simulink model "direction_sim"  (R2023a)
settings: configuration reference "config" (kept outside this file)
model workspace (MATLAB code in the model file + MAT data in the model file):
  cmdLim = Simulink.Parameter
  cmdLim.Value = 15
  cmdLim.Description = 'Limit for controlling the maximum surface command angle.'
  cmdLim.Min = 0
  cmdLim.Max = 90
  cmdLim.DocUnits = 'deg'
  dispGain = Simulink.Parameter
  dispGain.Value = 0.75
  dispGain.Description = 'Gain applied to the displacement error.'
  dispGain.Min = 0
  dispGain.Max = []
  dispGain.DocUnits = 'deg/sec/deg'
  dispLim = Simulink.Parameter
  dispLim.Value = 30
  dispLim.Description = 'Limit for controlling the maximum commanded angle.'
  dispLim.Min = 0
  dispLim.Max = 180
  dispLim.DocUnits = 'deg'
  intGain = Simulink.Parameter
  intGain.Value = 0.5
  intGain.Description = 'Gain applied to the integral error.'
  intGain.Min = 0
  intGain.Max = []
  intGain.DocUnits = 'deg/sec/deg/sec'
  intLim = Simulink.Parameter
  intLim.Value = 5
  intLim.Description = 'Limit for controlling the maximum commanded angle.'
  intLim.Min = 0
  intLim.Max = 90
  intLim.DocUnits = 'deg'
  rateGain = Simulink.Parameter
  rateGain.Value = 2
  rateGain.Description = 'Gain applied to the rate error.'
  rateGain.Min = 0
  rateGain.Max = []
  rateGain.DocUnits = 'deg/deg/sec'
  rateLim = Simulink.Parameter
  rateLim.Value = 6
  rateLim.Description = 'Limit for controlling the maximum commanded angle.'
  rateLim.Min = 0
  rateLim.Max = 180
  rateLim.DocUnits = 'deg/sec'
  hdgGain = Simulink.Parameter
  hdgGain.Value = 0.015
  b = Simulink.Parameter
  b.Value = 0.001
  b.DataType = 'single'
  b.Complexity = 'real'
  b.Dimensions = [1 1]
  enc_line = Simulink.Parameter
  enc_line.Value = 10000
  enc_line.DataType = 'single'
  enc_line.Complexity = 'real'
  enc_line.Dimensions = [1 1]
  fc = Simulink.Parameter
  fc.Value = 0.01
  fc.DataType = 'single'
  fc.Complexity = 'real'
  fc.Dimensions = [1 1]
  flux = Simulink.Parameter
  flux.Value = 0.0125
  flux.DataType = 'single'
  flux.Complexity = 'real'
  flux.Dimensions = [1 1]
  fs = Simulink.Parameter
  fs.Value = 10000
  fs.Description = '位置环 速度环执行频率'
  fs.DataType = 'single'
  fs.Complexity = 'real'
  fs.Dimensions = [1 1]
  j = Simulink.Parameter
  j.Value = 1.9e-05
  j.DataType = 'single'
  j.Complexity = 'real'
  j.Dimensions = [1 1]
  j_inv = Simulink.Parameter
  j_inv.Value = 52631.5789474
  j_inv.DataType = 'single'
  j_inv.Complexity = 'real'
  j_inv.Dimensions = [1 1]
  kt = Simulink.Parameter
  kt.Value = 0.075
  kt.DataType = 'single'
  kt.Complexity = 'real'
  kt.Dimensions = [1 1]
  ld = Simulink.Parameter
  ld.Value = 0.00059
  ld.Description = '定子电感 H'
  ld.DataType = 'single'
  ld.Complexity = 'real'
  ld.Dimensions = [1 1]
  ld_inv = Simulink.Parameter
  ld_inv.Value = 1694.91525424
  ld_inv.Description = '定子电感 H'
  ld_inv.DataType = 'single'
  ld_inv.Complexity = 'real'
  ld_inv.Dimensions = [1 1]
  lq = Simulink.Parameter
  lq.Value = 0.00059
  lq.Description = '定子电感 H'
  lq.DataType = 'single'
  lq.Complexity = 'real'
  lq.Dimensions = [1 1]
  lq_inv = Simulink.Parameter
  lq_inv.Value = 1694.91525424
  lq_inv.Description = '定子电感 H'
  lq_inv.DataType = 'single'
  lq_inv.Complexity = 'real'
  lq_inv.Dimensions = [1 1]
  pn = Simulink.Parameter
  pn.Value = 4
  pn.DataType = 'single'
  pn.Complexity = 'real'
  pn.Dimensions = [1 1]
  r = Simulink.Parameter
  r.Value = 1.02
  r.Description = '定子电阻 ohm'
  r.DataType = 'single'
  r.Complexity = 'real'
  r.Dimensions = [1 1]
  tc = Simulink.Parameter
  tc.Value = 5e-05
  tc.Description = '电流环运行频率用来设定综合仿真的参数'
  tc.DataType = 'double'
  tc.Complexity = 'real'
  tc.Dimensions = [1 1]
  tp = Simulink.Parameter
  tp.Value = 0.0001
  tp.Description = '位置环速度环执行周期'
  tp.DataType = 'double'
  tp.Complexity = 'real'
  tp.Dimensions = [1 1]
  ts = Simulink.Parameter
  ts.Value = 1e-05
  ts.Description = '模型仿真的周期 s'
  ts.DataType = 'double'
  ts.Complexity = 'real'
  ts.Dimensions = [1 1]
libraries: simulink x2
settings Model: RequirementInfo={} %GIDa_fe9045fd_0412_4b6e_8206_617cc20e6fde  DataDictionary=model_config.sldd  ParameterArgumentNames=b,enc_line,fc,flux,fs,j,j_inv,kt,ld,ld_inv,lq,lq_inv,pn,r  Creator=Administrator  LastModifiedBy=Administrator
settings ConfigSetRef: SourceName=config

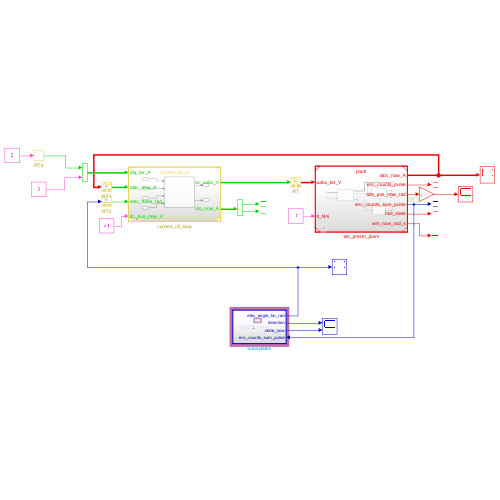
[thumbnail: Simulink's stored preview of the top-level diagram]
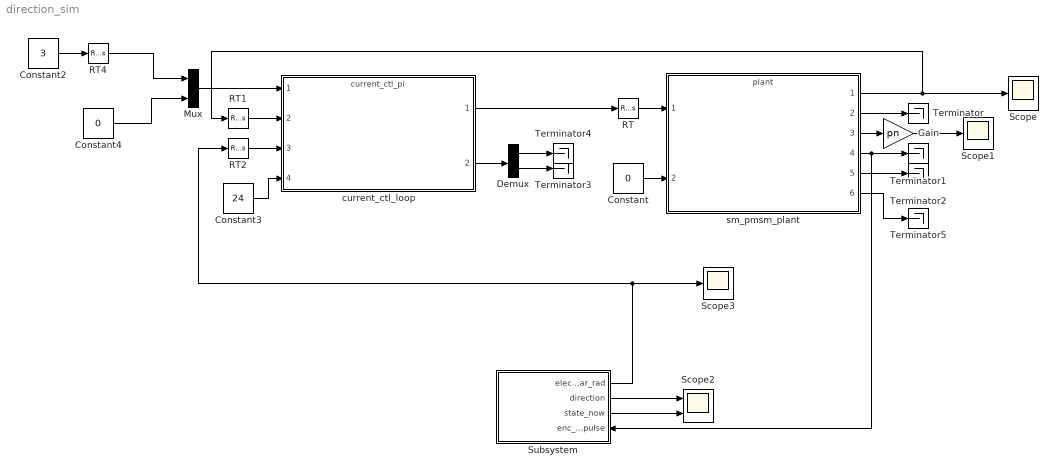
== system direction_sim ==
  Constant : Constant  Value=0  OutDataTypeStr=single
  Constant2 : Constant  Value=3  OutDataTypeStr=single
  Constant3 : Constant  Value=24  OutDataTypeStr=single
  Constant4 : Constant  Value=0  OutDataTypeStr=single
  Demux : Demux  Outputs=2
  Gain : Gain  Gain=pn
  Mux : Mux  Inputs=2
  RT : RateTransition  OutPortSampleTime=ts
  RT1 : RateTransition  OutPortSampleTime=tc
  RT2 : RateTransition  OutPortSampleTime=tc
  RT4 : RateTransition  OutPortSampleTime=tc
  Scope : Scope
  Scope1 : Scope
  Scope2 : Scope  NumInputPorts=2
  Scope3 : Scope
  Subsystem : Subsystem  TreatAsAtomicUnit=on  SystemSampleTime=10e-5
      settings: PortSchema="{\"entries\":[{\"content\":{\"sides\":[{\"content\":{},\"type\":\"ConnectorPlacement.EquallySpacedRectSide\",\"uuid\":\"d07efbd3-f561-406e-a8ff-2cd425a2d2f1\"},{\"content\":{\"connectorIds\":[\"Out1\",\"Out2\",\"Out3\",\"In1\"],\"side\":\"RIGHT\"},\"type\":\"ConnectorPlacement.EquallySpacedRectSide\",\"uuid\":\"8e75d4b6-33a0-42ab-8f9a-b924bdc8bdb3\"},{\"content\":{\"side\":\"TOP\"},\"type\":\"ConnectorPlacement.EquallySpacedRectSide\",\"uuid\":\"05e65f83-a04f-4767-afb8-de784f70a9b2\"}]},\"type\":\"ConnectorPlacement.EquallySpacedConnector\",\"uuid\":\"6847f190-d81b-4cfc-961e-3d73d3d3f65e\"}],\"packageUris\":[\"http://schema.mathworks.com/mf0/Connector/R2020b\"],\"version\":\"1.0\"}"
  Terminator{,1..5} (6 alike) : Terminator
  current_ctl_loop : ModelReference  ModelNameDialog=current_ctl_pi.slx  UsingDefaultArgumentValue=0,0,0,0,0,0,0,0,0  SimulationMode=Normal  ModelReferenceVersion=2.139
  sm_pmsm_plant : ModelReference  ModelNameDialog=plant.slx  UsingDefaultArgumentValue=0,0,0,0,0,0,0,0,0,0,0,0,0,0,0,0,0,0,0,0,0,0,0,0,0,0  SimulationMode=Normal  ModelReferenceVersion=1.25
  wires:
  Constant/1 -> sm_pmsm_plant/2
  current_ctl_loop/1 -> RT/1
  Mux/1 -> current_ctl_loop/1
  sm_pmsm_plant/3 -> Gain/1
  sm_pmsm_plant/2 -> Terminator/1
  sm_pmsm_plant/5 -> Terminator2/1
  RT/1 -> sm_pmsm_plant/1
  sm_pmsm_plant/1 -> RT1/1, Scope/1
  current_ctl_loop/2 -> Demux/1
  RT2/1 -> current_ctl_loop/3
  sm_pmsm_plant/4 -> Terminator1/1, Subsystem/1(enc_counts_sum_pulse)
  Demux/2 -> Terminator3/1
  RT1/1 -> current_ctl_loop/2
  Demux/1 -> Terminator4/1
  Constant3/1 -> current_ctl_loop/4
  sm_pmsm_plant/6 -> Terminator5/1
  RT4/1 -> Mux/1
  Constant4/1 -> Mux/2
  Constant2/1 -> RT4/1
  Gain/1 -> Scope1/1
  Subsystem/1(elec_angle_tar_rad) -> Scope3/1, RT2/1
  Subsystem/2(direction) -> Scope2/1
  Subsystem/3(state_now) -> Scope2/2

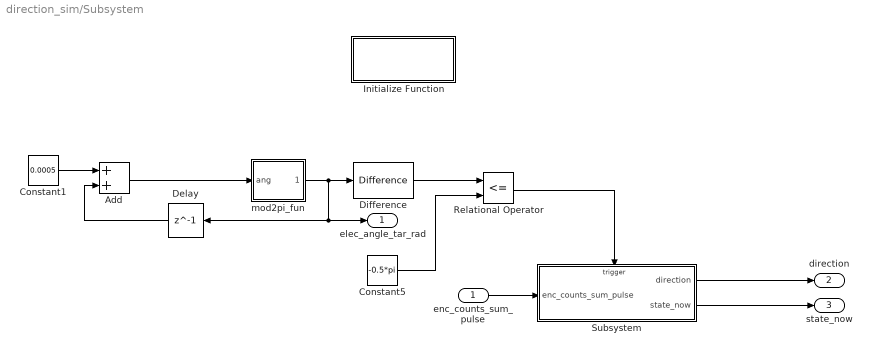
== system direction_sim/Subsystem ==
  enc_counts_sum_pulse : Inport
  Add : Sum
  Constant1 : Constant  Value=0.0005
  Constant5 : Constant  Value=-0.5*pi
  Delay : Delay  DelayLength=1
  Difference : simulink/Discrete/Difference  ICPrevInput=0.0  OutMin=[]  OutMax=[]  OutDataType=fixdt(1, 16)  OutScaling=2^-10  DoSatur=off
  Initialize Function : Subsystem  TreatAsAtomicUnit=on
  Relational Operator : RelationalOperator  Operator=<=  OutDataTypeStr=boolean  RndMeth=Simplest  InputSameDT=off
  Subsystem : Subsystem
  mod2pi_fun : MATLAB Function  TreatAsAtomicUnit=on
  elec_angle_tar_rad : Outport
  direction : Outport  Port=2
  state_now : Outport  Port=3
  wires:
  Constant1/1 -> Add/1
  Add/1 -> mod2pi_fun/1(ang)
  Difference/1 -> Relational Operator/1
  Delay/1 -> Add/2
  mod2pi_fun/1(n_ang) -> Delay/1, elec_angle_tar_rad/1, Difference/1
  enc_counts_sum_pulse/1 -> Subsystem/1(enc_counts_sum_pulse)
  Relational Operator/1 -> Subsystem/Trigger
  Constant5/1 -> Relational Operator/2
  Subsystem/1(direction) -> direction/1
  Subsystem/2(state_now) -> state_now/1

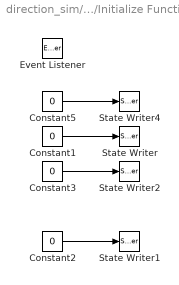
== system direction_sim/Subsystem/Initialize Function ==
  Constant1 : Constant  Value=0  OutDataTypeStr=single
  Constant2 : Constant  Value=0  OutDataTypeStr=single
  Constant3 : Constant  Value=0  OutDataTypeStr=int64
  Constant5 : Constant  Value=0  OutDataTypeStr=boolean
  Event Listener : EventListener  DisableCoverage=on  EventName=reset
  State Writer : StateWriter  StateOwnerBlock=../../Delay
  State Writer1 : StateWriter  StateOwnerBlock=../../Difference/UD
  State Writer2 : StateWriter  StateOwnerBlock=../../Subsystem/Difference/UD
  State Writer4 : StateWriter  StateOwnerBlock=../../Subsystem/Trigger
  wires:
  Constant5/1 -> State Writer4/1
  Constant1/1 -> State Writer/1
  Constant3/1 -> State Writer2/1
  Constant2/1 -> State Writer1/1

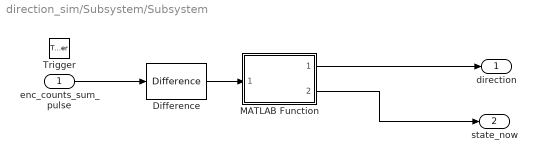
== system direction_sim/Subsystem/Subsystem ==
  enc_counts_sum_pulse : Inport
  Trigger : TriggerPort  VariantControl=(inherit)  PortDimensions=1
  Difference : simulink/Discrete/Difference  ICPrevInput=0.0  OutMin=[]  OutMax=[]  OutDataType=fixdt(1, 16)  OutScaling=2^-10  DoSatur=off
  MATLAB Function : MATLAB Function  TreatAsAtomicUnit=on
  direction : Outport
  state_now : Outport  Port=2
  wires:
  enc_counts_sum_pulse/1 -> Difference/1
  Difference/1 -> MATLAB Function/1(diff_pos)
  MATLAB Function/1(direction) -> direction/1
  MATLAB Function/2(state_now) -> state_now/1

== matlab function direction_sim/Subsystem/mod2pi_fun ==
  data: ang input; n_ang output
function n_ang = mod2pi(ang)
    % 将角度限制在0到2π范围内
    TWO_PI = single(2*pi);
    n_ang = single(ang);
    while n_ang < 0
        n_ang = n_ang + TWO_PI;
    end
    while n_ang >= TWO_PI
        n_ang = n_ang - TWO_PI;
    end
end

== matlab function direction_sim/Subsystem/Subsystem/MATLAB Function ==
  data: diff_pos input; direction output; state_now output
function [direction, state_now] = direction_id(diff_pos)

if diff_pos > 0
    direction = int8(1);
    state_now = int8(3);
elseif diff_pos < 0 
    direction = int8(-1);
    state_now = int8(3);
else
    direction = int8(0);
    state_now = int8(2);
end
